simulink model "Vehicle_Model_Controller_Mar16"  (R2020b)
settings: Solver=VariableStepAuto  StartTime=0.0  StopTime=20  FixedStep=0.015  MaxStep=0.015  RelTol=1e-3
model workspace (MAT data in the model file):
  Kp = 10
  understeer_gradient = 0.05
values from neighbouring files (symbols this model uses):
  I = 0    [startup.m]
  P = 10    [startup.m]
  T = 0    [startup.m]
undefined symbols (not defined in the file or in its folder): DiscIntNeverNeededParam
libraries: fl_lib x32, nesl_utility x24, sdl_lib x8, cstblocks x1, pid_lib x1, vehdynlibsteering x1, autolibshared x1, autolibdatasheetbattery x1
(part 3 of 3)

== matlab function Vehicle_Model_Controller_Mar16/Driver Input Logic/Torque Vectoring Controller/LP_Calc  ==
  settings: updateMethod=DISCRETE
  data: Tx_actual output double; driver_input input; power_limit_battery input; FY input; omega_m input; x input; y input; T2F input; slip_limit input; power_limit input; tau_limit_upper input; tau_limit_lower input; rpm_limit input; omega_m output; lb output single; PID input; ub output single; M_max output double; J_z data_store_memory; motor_efficiency data_store_memory; motor_limit_torque data_store_memory; min_speed_regen data_store_memory; power output double; bigM_flag output; typed output; zero_crossing output; yaw_accel output double
function [Tx_actual, omega_m, lb, ub, M_max, power, bigM_flag, typed, zero_crossing, yaw_accel] = LP_calc(driver_input, power_limit_battery, FY, omega_m, x, y, T2F, slip_limit, power_limit, tau_limit_upper, tau_limit_lower, rpm_limit, PID)
%% LP_calc Computation
% Developer(s):    David Farell
%                  Demetrius Gulewicz
%                  Elliot Stockwell
%                  Tao Sun
%
% Developed for: Purdue Electric Racing
% Date:          12/25/2021
%
% Description: This function primarily computes the desired torque
%              distribution after constructing an optimization statement.
%
%
%% Pass Through Signals
% omega_m - Motor Shaft Angular Velocity [rad/s][1x4]
%
%
%% Input Only
% prev_torque - Torque Requested To Motor In Previous Time Step [Nm][4x1]
% driver_input - Proportion of total available power to use [Unitless][1x1]
% T2F - Convert Torque At The Motor Shaft to Force At The Tire [1/m][1x4]
% power_limit_battery - Max & Min Total Battery Power Output [W][1x2]
% FY - Tires Forces y Direction, Tire fixed coordinates [N][1x4]
% x - Equivalent Distances That FX Acts From CoG [m][1x4]
% y - Equivalent Distances That FY Acts From CoG [m][1x4]
% slip_limit - Max Torque Before Tire Slips [Nm][1x4]
% torque_limit_motor - Max Torque Motor Can Output [Nm][1x4]
% tau_limit_upper - Max Torque Motor Is Allowed To Change To [Nm][1x4]
% tau_limit_lower - Min Torque Motor Is Allowed To Change To [Nm][1x4]
% PID - Desired Yaw Acceleration [rad/s^2][1x1]
%
%
%% Output Only
% Tx - Torque Request To Motors [Nm][4x1]
% lb - Min Torque Request [Nm][1x4]
% ub - Max Torque Request [Nm][1x4]
% Aeq - Moment About CoG, Optimization Variable [rad/s^2][1x1]
% beq - Moment About CoG, Yaw Acceleration & Other Foces [rad/s^2][1x1]
% A - Power Consumed, Optimization Variable [W][1x1]
% b - Power Consumed, Driver Input [W][1x1]
% M_max - Max & Min Yaw Acceleration Achievable With lb & ub [rad/s^2][1x2]
% Power - Total Estimated Power Consumed by the 4 Motors
% TR - The Estimated Yaw Acceleration from the Vehicle
%
%
%% Constants
global J_z; % Polar Moment Of Inertia [kg m^2][1x1]
global motor_efficiency; % Motor efficiency [Unitless][1x4]
global motor_limit_torque; % Minimum & Max Torque Request From Motor [Nm][1x2]
global min_speed_regen; % Min Motor Shaft Speed For Regen Braking [rad/s][1x1]


%% Calculation
% Calculate Boundary Conditions, The Max and Min Allowable Torque
ub = single([0, 0, 0, 0]);
lb = single([0, 0, 0, 0]);

slip_limit = single([50 50 50 50]);

for i = 1:4
    ub(i) = min([slip_limit(i), power_limit(i), motor_limit_torque(2), tau_limit_upper(i), rpm_limit(i)]);
    lb(i) = max([-slip_limit(i), -power_limit(i), motor_limit_torque(1), tau_limit_lower(i)]);
end

% Enforce No Backwards Rotation Of Tires
for i = 1:4
   if omega_m(i) < min_speed_regen && lb(i) < 0
       lb(i) = 0;
   end
end

% Max & Min Forces on the Tires
ub_f = ub .* T2F;
lb_f = lb .* T2F;

% Find Max & Min For PID, The Yaw Acceleration Of The Car
M_max=zeros(1,2);
M_max(1) = (x(1)*ub_f(1)+x(3)*ub_f(3)+x(2)*lb_f(2)+x(4)*lb_f(4)+sum(y.*FY))/J_z;
M_max(2) = (x(2)*ub_f(2)+x(4)*ub_f(4)+x(1)*lb_f(1)+x(3)*lb_f(3)+sum(y.*FY))/J_z;

% Limit PID To Be No Larger Than Possible Due To Torque Constraints
if PID >= M_max(1)
    PID = M_max(1);
elseif PID <= M_max(2)
    PID = M_max(2);
end

% Calculate Yaw Constraint
Aeq = ((1 ./ J_z) .* x) .* T2F;
beq = single(PID-sum(((1 / J_z) * y) .* FY));

if beq == 0
    beq = single(0.0000001);
end

%% Determine How to Optimize
if driver_input > 0
%     A = single([(omega_m ./ motor_efficiency); -(omega_m ./ motor_efficiency)]);
%     b = single([driver_input*power_limit_battery, 0]);
      A = single(omega_m ./ motor_efficiency);
      b = single(driver_input*power_limit_battery);
else 
%     A = single([-(omega_m ./ motor_efficiency); (omega_m ./ motor_efficiency)]);
%     b = single([driver_input*power_limit_battery, 0]);
      A = single(omega_m ./ motor_efficiency);
      b = single(driver_input*power_limit_battery);
end

%% Detect Potential Zero Crossing, Determine Augmented lb and ub
lb_plus = lb;
ub_neg = ub;
zero_crossing = 0;
crossing_locations = [0 0 0 0];
yaw_error_limit = (0.0002);

for i = 1:4
    if lb_plus(i) < 0 && ub_neg(i) > 0 
        lb_plus(i) = 0.001;
        ub_neg(i) = -0.001;
        zero_crossing = 1;
        crossing_locations(i) = i;
    end
end

signs_lb = sign(lb_plus);
signs_ub = sign(ub_neg);
signs = sign(lb);
             
%% Optimization
Tx = single([0 0 0 0]);
bigM_flag = single(0);
typed = 0;
ub_adjust = [0 0 0 0];
lb_adjust = [0 0 0 0];
signs_adust = [0 0 0 0];

if driver_input >= 0
    if zero_crossing == 1 && omega_m(1) > 10    
            [Tx31, Tx32, Tx33, Tx34, bigM_flag3] = call_bigM_C(T2F, b, A, beq, Aeq, lb, ub_neg, signs_ub, yaw_error_limit*1000);           
            Tx3 = double([Tx31, Tx32, Tx33, Tx34]);
            
            for i = 1:4
                if abs(Tx3(i)) < 0.002 && crossing_locations(i) > 0
                    lb_adjust(i) = lb_plus(i);
                    ub_adjust(i) = ub(i);
                else
                    lb_adjust(i) = lb(i);
                    ub_adjust(i) = ub(i);
                end
            end
            
            signs_adust = sign(lb_adjust);
            [Tx21, Tx22, Tx23, Tx24, bigM_flag2] = call_bigM_C(T2F, b, A, beq, Aeq, lb_adjust, ub_adjust, signs_adust, yaw_error_limit*1000);
            Tx2 = double([Tx21, Tx22, Tx23, Tx24]);
            
            if bigM_flag2 == 1 || bigM_flag2 == 3 || bigM_flag3 == 1 || bigM_flag3 == 3
                Tx = single(Tx2);
                typed = 2;
                bigM_flag = single(bigM_flag2);
            else
                [Tx5, bigM_flag5] = call_bigM_alt(b, A, beq, Aeq, lb_plus, ub);
                [Tx6, bigM_flag6] = call_bigM_alt(b, A, beq, Aeq, lb, ub_neg);

                if sum(abs(Tx5)) > sum(abs(Tx6))
                    Tx = single(Tx5);
                    typed = 5;
                    bigM_flag = single(bigM_flag5);
                else
                    Tx = single(Tx6);
                    typed = 6;
                    bigM_flag = single(bigM_flag6);
                end

            end
    else    
        [Tx11, Tx12, Tx13, Tx14, bigM_flag14] = call_bigM_C(T2F, b, A, beq, Aeq, lb, ub, signs, 0.05);
        Tx1 = [Tx11, Tx12, Tx13, Tx14];

        bigM_flag1 = single(bigM_flag14);
        
        if bigM_flag1 == 3 || bigM_flag1 == 1
            Tx = single(Tx1);
            typed = 1;
            bigM_flag = single(bigM_flag1);
        else
            [Tx4, bigM_flag4] = call_bigM_alt(b, A, beq, Aeq, lb, ub);
            bigM_flag = single(bigM_flag4);

            if bigM_flag4 == 3 || bigM_flag4 == 1
                Tx = single(Tx4);
                typed = 4;
                bigM_flag = single(bigM_flag4);
            end
        end   
    end
else
    if zero_crossing == 1 && omega_m(1) > 10
            [Tx2, bigM_flag2] = call_bigMz_brake(T2F, b, A, beq, Aeq, lb_plus, ub);
            [Tx3, bigM_flag3] = call_bigMz_brake(T2F, b, A, beq, Aeq, lb, ub_neg);

            if (bigM_flag2 == 3 || bigM_flag2 == 1) || (bigM_flag3 == 3 || bigM_flag3 == 1)
                if sum(abs(Tx2)) > sum(abs(Tx3))
                    Tx = single(Tx2);
                    typed = 2;
                    bigM_flag = single(bigM_flag2);
                else
                    Tx = single(Tx3);
                    typed = 3;
                    bigM_flag = single(bigM_flag3);
                end  
            else
                [Tx5, bigM_flag5] = call_bigM_alt(b, A, beq, Aeq, lb_plus, ub);
                [Tx6, bigM_flag6] = call_bigM_alt(b, A, beq, Aeq, lb, ub_neg);

                if sum(abs(Tx5)) > sum(abs(Tx6))
                    Tx = single(Tx5);
                    typed = 5;
                    bigM_flag = single(bigM_flag5);
                else
                    Tx = single(Tx6);
                    typed = 6;
                    bigM_flag = single(bigM_flag6);
                end

            end
    else
        [Tx1, bigM_flag1] = call_bigMz_brake(T2F, b, A, beq, Aeq, lb, ub);
        bigM_flag = single(bigM_flag1);

        if bigM_flag1 == 3 || bigM_flag1 == 1
            Tx = single(Tx1);
            typed = 1;
            bigM_flag = single(bigM_flag1);
        else
            [Tx4, bigM_flag4] = call_bigM_alt(b, A, beq, Aeq, lb, ub);
            bigM_flag = single(bigM_flag4);

            if bigM_flag4 == 3 || bigM_flag4 == 1
                Tx = single(Tx4);
                typed = 4;
                bigM_flag = single(bigM_flag4);
            end
        end   
    end
end

Tx_actual = double(Tx');
yaw_accel = double((sum(x.*T2F.*Tx_actual')+sum(y.*FY))/J_z);
power = double(sum(Tx_actual' .* omega_m));

end

== matlab function Vehicle_Model_Controller_Mar16/Motor and Battery/Motors/   ==
  data: Battery_Voltage input; ang_vel_RAD input; battery_current output; Motor_torque input; battery_power output
function [battery_current, battery_power]= get_batt_curr(Battery_Voltage, ang_vel_RAD, Motor_torque)
%% Current Draw
% Developers:    Demetrius Gulewicz

% Developed for: Purdue Electric Racing
% Date:          09/18/2021
%
% Definitions:
% ang_vel_RAD:   Angular velocity of each wheel on the wheel fixed y axis [RAD]
% Motor_torque:  Torque the motor actually outputs                 [Ncm]
% Battery_Voltage: The voltage of the battery                      [V]

%% Definitions
a = 0.0411;
b = 2.7976;
c = 45.978;

t = Motor_torque;
w = ang_vel_RAD;
v = Battery_Voltage;

e = 85;

%% Calculate Current Draw
%x0 = [20, 20, 20, 20];
%options = optimoptions('fsolve','Algorithm','Levenberg-Marquardt');
%F = @(x) ([(a * x(1)^3) + (b * x(1)^2) + (c * x(1)), ] .* v) - (t .* w);
%battery_current = sum(fsolve(F,x0,options));

battery_current = sum((t .* w') ./ (e .* v));
battery_power = battery_current * Battery_Voltage;
end
